simulink model "lab5_2"  (R2018b)
settings: Solver=FixedStepAuto  StartTime=0.0  StopTime=2.0  RelTol=1e-3
libraries: roblocks x3
settings Model: Creator=asset.rayev  LastModifiedBy=asset.rayev

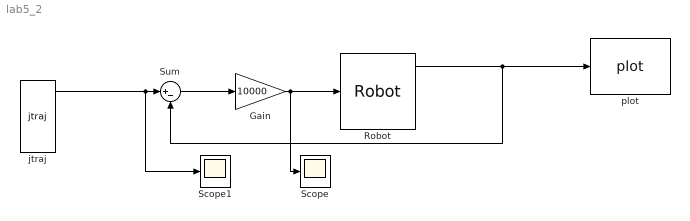
== system lab5_2 ==
  Gain : Gain  Gain=10000
  Robot : roblocks/Arm/Robot  robot=chappy  q0=[0 0 0]
  Scope : Scope
  Scope1 : Scope
  Sum : Sum  Inputs=|+-
  jtraj : roblocks/Toolbox/jtraj  q0=[0 0 0]  qf=[pi/2 -pi/4 -pi/4]  tmax=2  ts=0.02
  plot : roblocks/Arm/plot  robot=chappy  fps=5  holdplot=on
  wires:
  jtraj/1 -> Scope1/1, Sum/1
  Sum/1 -> Gain/1
  Gain/1 -> Scope/1, Robot/1
  Robot/1 -> Sum/2, plot/1
